simulink model "Linear_Moving_Setpoint_SS_Integral"  (R2020b)
settings: Solver=VariableStepAuto  StartTime=0.0  StopTime=t_sim  RelTol=1e-9
undefined symbols (not defined in the file): A1a_sim, B1a_sim, C1a_setp_ctrl, des_traj_handle, K1a, r_sim, S1a_sim, SP_sel, x1a_0
settings Model: Creator=domin  LastModifiedBy=domin

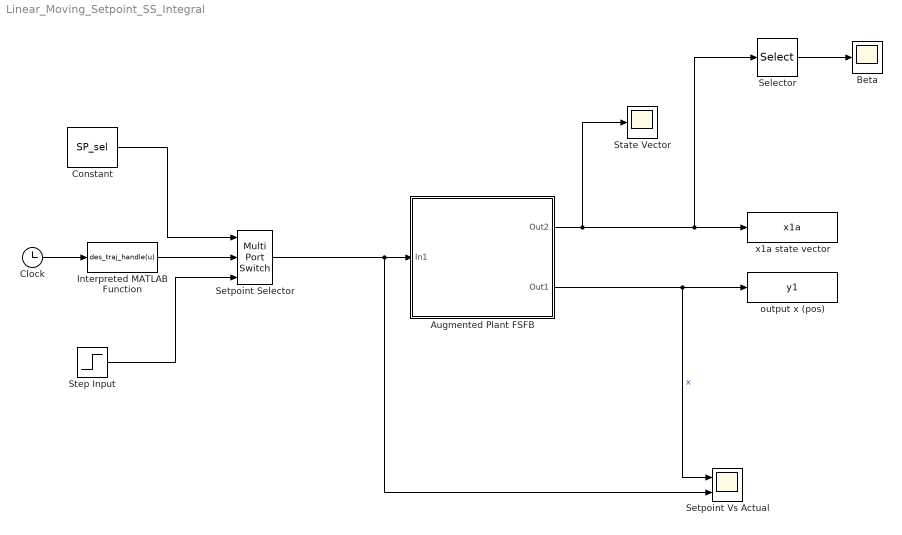
== system Linear_Moving_Setpoint_SS_Integral ==
  Augmented Plant FSFB : Subsystem
  Beta : Scope
  Clock : Clock
  Constant : Constant  Value=SP_sel
  Interpreted MATLAB Function : MATLABFcn  MATLABFcn=des_traj_handle(u)
  Selector : Selector  InputPortWidth=5  IndexOptions=Index vector (dialog)  Indices=[2]  OutputSizes=1
  Setpoint Selector : MultiPortSwitch  Inputs=2
  Setpoint Vs Actual : Scope  NumInputPorts=2
  State Vector : Scope
  Step Input : Step  After=r_sim  SampleTime=0
  output x (pos) : ToWorkspace  VariableName=y1  SampleTime=-1
  x1a state vector : ToWorkspace  VariableName=x1a  SampleTime=-1
  wires:
  Setpoint Selector/1 -> Setpoint Vs Actual/2, Augmented Plant FSFB/1(In1)
  Augmented Plant FSFB/2(Out1) -> Setpoint Vs Actual/1, output x (pos)/1  "x"
  Augmented Plant FSFB/1(Out2) -> Selector/1, x1a state vector/1, State Vector/1
  Interpreted MATLAB Function/1 -> Setpoint Selector/2
  Step Input/1 -> Setpoint Selector/3
  Constant/1 -> Setpoint Selector/1
  Clock/1 -> Interpreted MATLAB Function/1
  Selector/1 -> Beta/1

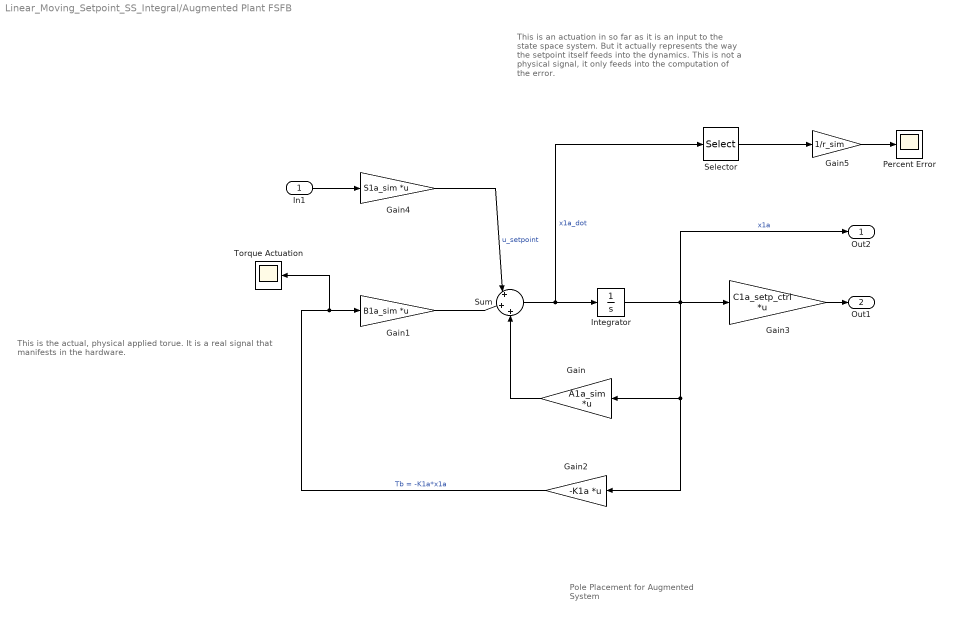
== system Linear_Moving_Setpoint_SS_Integral/Augmented Plant FSFB ==
  note: This is the actual, physical applied torue. It is a real signal
      | that manifests in the hardware.
  note: This is an actuation in so far as it is an input to the
      | state space system. But it actually represents the
      | way the setpoint itself feeds into the dynamics. This
      | is not a physical signal, it only feeds into the
      | computation of the error.
  note: Pole Placement for
      | Augmented System
  In1 : Inport
  Gain : Gain  Gain=A1a_sim  Multiplication=Matrix(K*u)
  Gain1 : Gain  Gain=B1a_sim  Multiplication=Matrix(K*u)
  Gain2 : Gain  Gain=-K1a  Multiplication=Matrix(K*u)
  Gain3 : Gain  Gain=C1a_setp_ctrl  Multiplication=Matrix(K*u)
  Gain4 : Gain  Gain=S1a_sim  Multiplication=Matrix(K*u)
  Gain5 : Gain  Gain=1/r_sim
  Integrator : Integrator  InitialCondition=x1a_0
  Percent Error : Scope
  Selector : Selector  InputPortWidth=5  IndexOptions=Index vector (dialog)  Indices=[5]  OutputSizes=1
  Sum : Sum  Inputs=|+|+|+
  Torque Actuation : Scope
  Out2 : Outport
  Out1 : Outport  Port=2
  wires:
  Gain1/1 -> Sum/2
  Sum/1 -> Selector/1, Integrator/1  "x1a_dot"
  Integrator/1 -> Out2/1, Gain2/1, Gain/1, Gain3/1  "x1a"
  Gain3/1 -> Out1/1
  Gain/1 -> Sum/3
  Gain2/1 -> Torque Actuation/1, Gain1/1  "Tb = -K1a*x1a"
  In1/1 -> Gain4/1
  Gain4/1 -> Sum/1  "u_setpoint"
  Gain5/1 -> Percent Error/1
  Selector/1 -> Gain5/1
